simulink model "Model_2_SpeedClosedLoop"  (R2025a)
settings: Solver=VariableStepAuto  StartTime=0.0  StopTime=3  MaxStep=1e-4  RelTol=1e-3  EnableMultiTasking=on
undefined symbols (not defined in the file): Gain_I, Gain_P, Lambda_m, Ld, Lq, Polepairs, Rs, Speed_Gain_I, Speed_Gain_P
libraries: spsControlledVoltageSourceLib x3, slpidlib x3, spsPermanentMagnetSynchronousMachineLib x1, spsGroundLib x1, SignalEditorBlockLib x1, spspowerguiLib x1
settings Model: Creator=dakaihu  LastModifiedBy=ernes
settings SolverCC: AlgebraicLoopSolver=TrustRegion
settings DataIOCC: LimitDataPoints=on  ReturnWorkspaceOutputsName=SDOSimTest_Log
settings OptimizationCC: LifeSpan=inf
settings DebuggingCC: UnconnectedInputMsg=warning  UnconnectedOutputMsg=warning  UnconnectedLineMsg=warning  AllowSymbolicDim=off  SFUnexpectedBacktrackingDiag=warning  SFNoUnconditionalDefaultTransitionDiag=warning  SFExecutionAtInitializationDiag=none  ArithmeticOperatorsInVariantConditions=warning
settings ModelReferenceCC: EnableRefExpFcnMdlSchedulingChecks=on  PropagateSignalLabelsOutOfModel=off
settings SFSimCC: SimUseLocalCustomCode=off  CustomCodeUndefinedFunction=UseInterfaceOnly
settings RTWCC: RTWUseLocalCustomCode=off  GPUComputeCapability=3.5
settings CodeAppCC: StateflowObjectComments=on
settings GRTTargetCC: TargetLangStandard=C89/C90 (ANSI)
settings ConfigComp: CovMetricSettings=dw  CovSaveCumulativeToWorkspaceVar=on  CovSaveSingleToWorkspaceVar=on  CovExternalEMLEnable=off
settings SimscapeCC: SimscapeNormalizeSystem=off

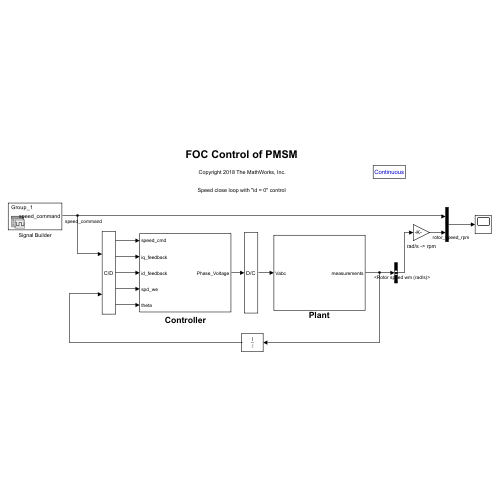
[thumbnail: Simulink's stored preview of the top-level diagram]
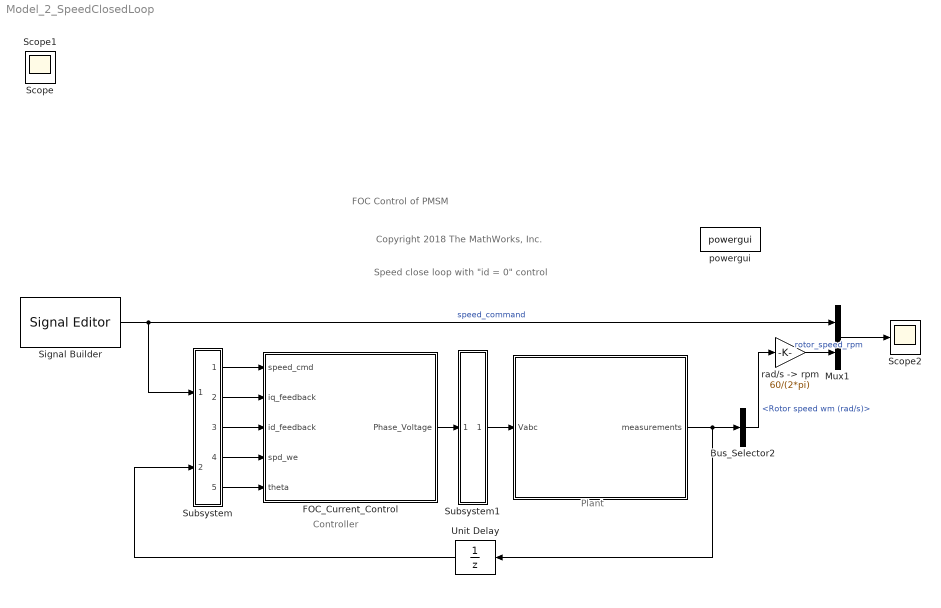
== system Model_2_SpeedClosedLoop ==
  note: Copyright 2018 The MathWorks, Inc.
  note: Speed close loop with "id = 0" control
  note: Controller
  note: Plant
  note: FOC Control of PMSM
  " " : Subsystem
  Bus_Selector2 : BusSelector  OutputSignals=Rotor speed wm (rad/s)
  FOC_Current_Control : Subsystem
  Mux1 : Mux  Inputs=2
  Scope2 : Scope
      settings: ActiveDisplayYMinimum=-125.56583  ActiveDisplayYMaximum=1130.09248
  Signal Builder : SignalEditorBlockLib/Signal Editor  FileName=SignalBuilder.mat  ActiveScenario=Group_1  ActiveSignal=speed_command  IsBus=off  OutputBusObjectStr=Bus: BusObject  SampleTime=0  OutputAfterFinalValue=Extrapolation  Unit=inherit  PreserveSignalName=on  ApplySigPropsToAllScenarios=on  ApplySigPropsToAllSignals=off  SignalPropertySource=Dialog parameters
  Subsystem : Subsystem
      mask Display: fprintf('C/D')
  Subsystem1 : Subsystem
      mask Display: fprintf('D/C')
  Unit Delay : UnitDelay  SampleTime=-1  HasFrameUpgradeWarning=on
  powergui : spspowerguiLib/powergui  SimulationMode=Continuous  SampleTime=1e-5  frequency=60  Iterations=50  frequencyindice=0  Pbase=100e6  ErrMax=1e-4  UnitsV=kV  UnitsW=MW  buscounter=0  FunctionMessages=off  echomessages=off  EnableUseOfTLC=off  CurrentSourceSwitches=off  DisableSnubberDevices=off  DisableRonSwitches=off  DisableVfSwitches=off  DisplayEquations=off  AutomaticDiscreteSolvers=off  SolverType=Tustin/Backward Euler (TBE)  Interpol=off  ExternalGateDelay=off  methode=off  Ts=100  x0status=blocks  SPID=on  SwTol=0  HookPort=off  NonlinearTolerance=1e-4  nMaxIteration=100  ContinueOnMaxIteration=off  RestoreLinks=warning  ResistiveCurrentMeasurement=off  Frange=[0:2:500]  Ylog=off  Xlog=on  ShowGrid=off  save=off  variable=ZData  structure=0  ZoomFFT=on  StartTime=0.0  cycles=1  DisplayStyle=1  fundamental=60  FreqAxis=off  MaxFrequency=1000  frequencyindicesteady=1  RmsSteady=1  display=off
  "rad/s -> rpm" : Gain  Gain=60/(2*pi)
  Scope : Scope
      settings: ActiveDisplayYMinimum=0.10553  ActiveDisplayYMaximum=0.2838
  Scope1 : Scope
      settings: ActiveDisplayYMinimum=-0.03595  ActiveDisplayYMaximum=0.48049  DataLoggingVariableName=ScopeData2
  wires:
  FOC_Current_Control/1(Phase_Voltage) -> Subsystem1/1(In1)
  " "/1(measurements) -> Unit Delay/1, Bus_Selector2/1
  Subsystem1/1(Out1) -> " "/1(Vabc)
  Unit Delay/1 -> Subsystem/2(PMSM_Measurements)
  Signal Builder/1 -> Subsystem/1(speed_cmd), Mux1/1  "speed_command"
  Subsystem/1(Out6) -> FOC_Current_Control/1(speed_cmd)
  Subsystem/2(Out2) -> FOC_Current_Control/2(iq_feedback)
  Subsystem/3(Out3) -> FOC_Current_Control/3(id_feedback)
  Subsystem/4(Out1) -> FOC_Current_Control/4(spd_we)
  Subsystem/5(Out4) -> FOC_Current_Control/5(theta)
  Bus_Selector2/1 -> "rad/s -> rpm"/1  "<Rotor speed wm (rad/s)>"
  "rad/s -> rpm"/1 -> Mux1/2  "rotor_speed_rpm"
  Mux1/1 -> Scope2/1

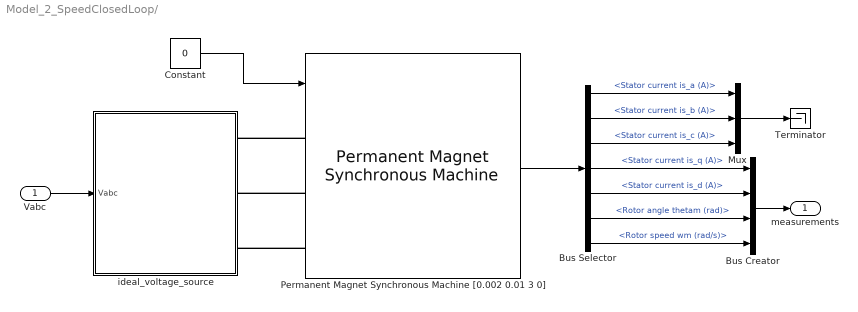
== system Model_2_SpeedClosedLoop/  ==
  Vabc : Inport
  Bus Creator : BusCreator  Inputs=4
  Bus Selector : BusSelector  OutputSignals=Stator current is_a (A),Stator current is_b (A),Stator current is_c (A),Stator current is_q (A),Stator current is_d (A),Rotor angle thetam (rad),Rotor speed wm (rad/s)
  Constant : Constant  Value=0
  Mux : Mux  Inputs=3
  Permanent Magnet Synchronous Machine [0.002 0.01 3 0] : spsPermanentMagnetSynchronousMachineLib/Permanent Magnet Synchronous Machine  NbPhases=3  FluxDistribution=Sinusoidal  RotorType=Salient-pole  MechanicalLoad=Torque Tm  PresetModel=No  ShowDetailedParameters=on  MeasurementBus=off  Resistance=Rs  Inductance=8.5e-3  dqInductances=[Ld,Lq]  La=0.000395  MachineConstant=Flux linkage established by magnets (V.s)  Flux=Lambda_m  VoltageCst=159.9771  TorqueCst=1.323  Flat=120  Mechanical=[0.0027 0.001 4 0]  PolePairs=Polepairs  InitialConditions=[0,0, 0,0]  InitialConditions5ph=[0 0 0 0 0 0]  RefAngle=Aligned with phase A axis (original Park)  IterativeDiscreteModel=Trapezoidal non iterative  TsBlock=-1  TsPowergui=0
  Terminator : Terminator
  ideal_voltage_source : Subsystem  VariantControl=variantPwm == enumPwm.behavior
  measurements : Outport  VectorParamsAs1DForOutWhenUnconnected=off
  wires:
  Vabc/1 -> ideal_voltage_source/1(Vabc)
  Bus Selector/4 -> Bus Creator/1  "<Stator current is_q (A)>"
  Bus Selector/5 -> Bus Creator/2  "<Stator current is_d (A)>"
  Bus Selector/6 -> Bus Creator/3  "<Rotor angle thetam (rad)>"
  Bus Creator/1 -> measurements/1
  Bus Selector/1 -> Mux/1  "<Stator current is_a (A)>"
  Bus Selector/2 -> Mux/2  "<Stator current is_b (A)>"
  Bus Selector/3 -> Mux/3  "<Stator current is_c (A)>"
  Mux/1 -> Terminator/1
  Permanent Magnet Synchronous Machine [0.002 0.01 3 0]/1 -> Bus Selector/1
  Bus Selector/7 -> Bus Creator/4  "<Rotor speed wm (rad/s)>"
  Constant/1 -> Permanent Magnet Synchronous Machine [0.002 0.01 3 0]/1
  connections:
  Permanent Magnet Synchronous Machine [0.002 0.01 3 0]/LConn1 -- ideal_voltage_source/RConn1
  Permanent Magnet Synchronous Machine [0.002 0.01 3 0]/LConn2 -- ideal_voltage_source/RConn2
  Permanent Magnet Synchronous Machine [0.002 0.01 3 0]/LConn3 -- ideal_voltage_source/RConn3

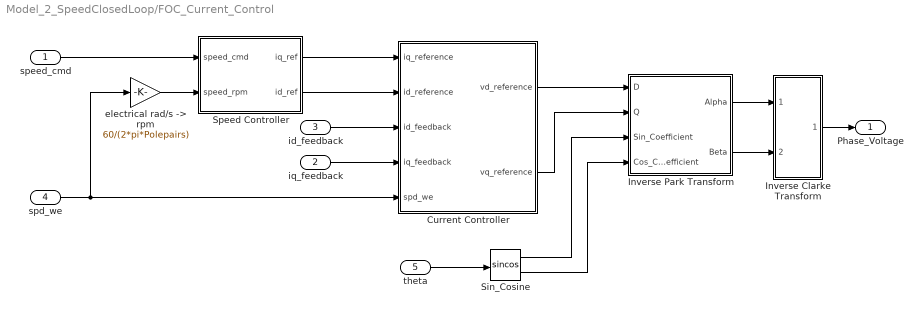
== system Model_2_SpeedClosedLoop/FOC_Current_Control ==
  speed_cmd : Inport
  iq_feedback : Inport  Port=2  SampleTime=1e-4
  id_feedback : Inport  Port=3  SampleTime=1e-4
  spd_we : Inport  Port=4
  theta : Inport  Port=5  SampleTime=1e-4
  Current Controller : Subsystem
  Inverse Clarke Transform : Subsystem
  Inverse Park Transform : Subsystem
  Sin_Cosine : Trigonometry  Operator=sincos
  Speed Controller : Subsystem
  "electrical rad/s -> rpm" : Gain  Gain=60/(2*pi*Polepairs)
  Phase_Voltage : Outport  SampleTime=1e-4  VectorParamsAs1DForOutWhenUnconnected=off
  wires:
  Inverse Clarke Transform/1(ABC) -> Phase_Voltage/1
  Sin_Cosine/2 -> Inverse Park Transform/4(Cos_Coefficient)
  Sin_Cosine/1 -> Inverse Park Transform/3(Sin_Coefficient)
  theta/1 -> Sin_Cosine/1
  Current Controller/2(vq_reference) -> Inverse Park Transform/2(Q)
  Current Controller/1(vd_reference) -> Inverse Park Transform/1(D)
  Inverse Park Transform/1(Alpha) -> Inverse Clarke Transform/1(Alpha)
  Inverse Park Transform/2(Beta) -> Inverse Clarke Transform/2(Beta)
  Speed Controller/1(iq_ref) -> Current Controller/1(iq_reference)
  Speed Controller/2(id_ref) -> Current Controller/2(id_reference)
  id_feedback/1 -> Current Controller/3(id_feedback)
  iq_feedback/1 -> Current Controller/4(iq_feedback)
  spd_we/1 -> "electrical rad/s -> rpm"/1, Current Controller/5(spd_we)
  "electrical rad/s -> rpm"/1 -> Speed Controller/2(speed_rpm)
  speed_cmd/1 -> Speed Controller/1(speed_cmd)

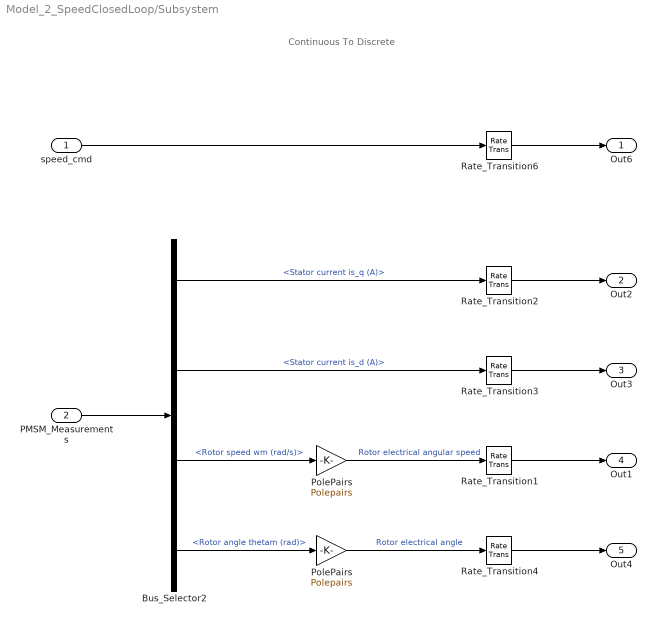
== system Model_2_SpeedClosedLoop/Subsystem ==
  note: Continuous To Discrete
  speed_cmd : Inport
  PMSM_Measurements : Inport  Port=2
  Bus_Selector2 : BusSelector  OutputSignals=Stator current is_q (A),Stator current is_d (A),Rotor speed wm (rad/s),Rotor angle thetam (rad)
  PolePairs : Gain  Gain=Polepairs
  "PolePairs " : Gain  Gain=Polepairs
  Rate_Transition{1..4,6} (5 alike) : RateTransition  Integrity=off  Deterministic=off
  Out6 : Outport  VectorParamsAs1DForOutWhenUnconnected=off
  Out2 : Outport  Port=2  VectorParamsAs1DForOutWhenUnconnected=off
  Out3 : Outport  Port=3  VectorParamsAs1DForOutWhenUnconnected=off
  Out1 : Outport  Port=4  VectorParamsAs1DForOutWhenUnconnected=off
  Out4 : Outport  Port=5  VectorParamsAs1DForOutWhenUnconnected=off
  wires:
  Rate_Transition4/1 -> Out4/1
  Bus_Selector2/2 -> Rate_Transition3/1  "<Stator current is_d (A)>"
  speed_cmd/1 -> Rate_Transition6/1
  Bus_Selector2/1 -> Rate_Transition2/1  "<Stator current is_q (A)>"
  Bus_Selector2/4 -> PolePairs/1  "<Rotor angle thetam (rad)>"
  PMSM_Measurements/1 -> Bus_Selector2/1
  PolePairs/1 -> Rate_Transition4/1  "Rotor electrical angle"
  Rate_Transition6/1 -> Out6/1
  Rate_Transition2/1 -> Out2/1
  Rate_Transition3/1 -> Out3/1
  Rate_Transition1/1 -> Out1/1
  Bus_Selector2/3 -> "PolePairs "/1  "<Rotor speed wm (rad/s)>"
  "PolePairs "/1 -> Rate_Transition1/1  "Rotor electrical angular speed"

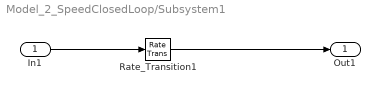
== system Model_2_SpeedClosedLoop/Subsystem1 ==
  In1 : Inport
  Rate_Transition1 : RateTransition  Integrity=off
  Out1 : Outport  VectorParamsAs1DForOutWhenUnconnected=off
  wires:
  In1/1 -> Rate_Transition1/1
  Rate_Transition1/1 -> Out1/1

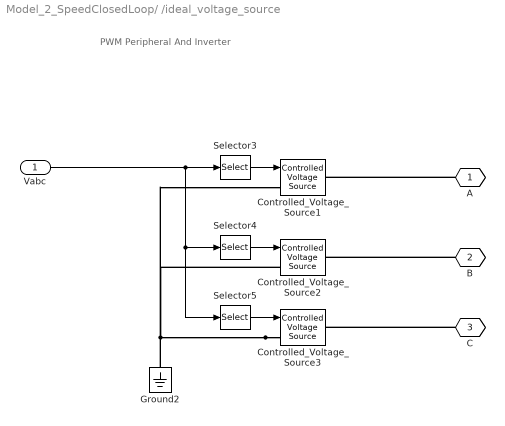
== system Model_2_SpeedClosedLoop/ /ideal_voltage_source ==
  note: PWM Peripheral And Inverter
  Vabc : Inport
  Controlled_Voltage_Source1 : spsControlledVoltageSourceLib/Controlled Voltage Source  Initialize=off  Source_Type=DC  Amplitude=12  Phase=0  Frequency=0  Measurements=None
  Controlled_Voltage_Source2 : spsControlledVoltageSourceLib/Controlled Voltage Source  Initialize=off  Source_Type=DC  Amplitude=12  Phase=0  Frequency=0  Measurements=None
  Controlled_Voltage_Source3 : spsControlledVoltageSourceLib/Controlled Voltage Source  Initialize=off  Source_Type=DC  Amplitude=12  Phase=0  Frequency=0  Measurements=None
  Ground2 : spsGroundLib/Ground  LConnTagsString=a
  Selector3 : Selector  InputPortWidth=3  IndexOptions=Index vector (dialog)  Indices=[1]  OutputSizes=1
  Selector4 : Selector  InputPortWidth=3  IndexOptions=Index vector (dialog)  Indices=2  OutputSizes=1
  Selector5 : Selector  InputPortWidth=3  IndexOptions=Index vector (dialog)  Indices=3  OutputSizes=1
  A : PMIOPort  Tag=PMCPort  Side=Right
  B : PMIOPort  Tag=PMCPort  Port=2  Side=Right
  C : PMIOPort  Tag=PMCPort  Port=3  Side=Right
  wires:
  Vabc/1 -> Selector4/1, Selector5/1, Selector3/1
  Selector5/1 -> Controlled_Voltage_Source3/1
  Selector4/1 -> Controlled_Voltage_Source2/1
  Selector3/1 -> Controlled_Voltage_Source1/1
  connections:
  C/RConn1 -- Controlled_Voltage_Source3/RConn1
  B/RConn1 -- Controlled_Voltage_Source2/RConn1
  A/RConn1 -- Controlled_Voltage_Source1/RConn1
  Controlled_Voltage_Source3/LConn1 -- Controlled_Voltage_Source1/LConn1 -- Controlled_Voltage_Source2/LConn1 -- Ground2/LConn1

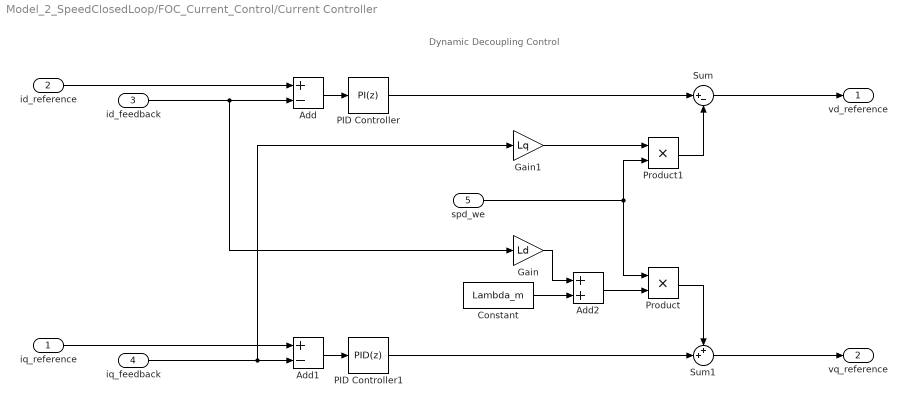
== system Model_2_SpeedClosedLoop/FOC_Current_Control/Current Controller ==
  note: Dynamic Decoupling Control
  iq_reference : Inport  SampleTime=1e-4
  id_reference : Inport  Port=2  SampleTime=1e-4
  id_feedback : Inport  Port=3  SampleTime=1e-4
  iq_feedback : Inport  Port=4  SampleTime=1e-4
  spd_we : Inport  Port=5  SampleTime=1e-4
  Add : Sum  Inputs=+-
  Add1 : Sum  Inputs=+-
  Add2 : Sum
  Constant : Constant  Value=Lambda_m  SampleTime=1e-4
  Gain : Gain  Gain=Ld
  Gain1 : Gain  Gain=Lq
  PID Controller : slpidlib/PID Controller  Controller=PI  Form=Parallel  TimeDomain=Discrete-time  UseExternalTs=off  SampleTime=-1  IntegratorMethod=Forward Euler  FilterMethod=Forward Euler  ControllerParametersSource=internal  P=Gain_P  I=Gain_I  UseKiTs=off  D=0  UseExternalDerivativeSource=off  N=100  UseFilter=on  TunerSelectOption=Transfer Function Based (PID Tuner App)  InitialConditionSource=internal  InitialConditionForIntegrator=0  InitialConditionForFilter=0  DifferentiatorICPrevScaledInput=0  ExternalReset=none  TrackingMode=off  Kt=1  LimitOutput=off  SatLimitsSource=internal  UpperSaturationLimit=inf  LowerSaturationLimit=-inf  LinearizeAsGain=on  AntiWindupMode=none  Kb=1  LimitIntegrator=off  UpperIntegratorSaturationLimit=inf  LowerIntegratorSaturationLimit=-inf  POutMin=[]  POutMax=[]  IOutMin=[]  IOutMax=[]  DOutMin=[]  DOutMax=[]  NOutMin=[]  NOutMax=[]  SumOutMin=[]  SumOutMax=[]  SaturationOutMin=[]  SaturationOutMax=[]  PParamMin=[]  PParamMax=[]  IParamMin=[]  IParamMax=[]  DParamMin=[]  DParamMax=[]  NParamMin=[]  NParamMax=[]  KbParamMin=[]  KbParamMax=[]  KtParamMin=[]  KtParamMax=[]  KbOutMin=[]  KbOutMax=[]  KtOutMin=[]  KtOutMax=[]  IntegratorOutMin=[]  IntegratorOutMax=[]  FilterOutMin=[]  FilterOutMax=[]  SumI1OutMin=[]  SumI1OutMax=[]  SumI2OutMin=[]  SumI2OutMax=[]  SumI3OutMin=[]  SumI3OutMax=[]  SumI4OutMin=[]  SumI4OutMax=[]  SumDOutMin=[]  SumDOutMax=[]  DifferentiatorOutMin=[]  DifferentiatorOutMax=[]  FilterDiffOutCoefMin=[]  FilterDiffOutCoefMax=[]  ReciprocalOutMin=[]  ReciprocalOutMax=[]  SumDenOutMin=[]  SumDenOutMax=[]  SumNumOutMin=[]  SumNumOutMax=[]  DivideOutMin=[]  DivideOutMax=[]  UdiffTsProdOutMin=[]  UdiffTsProdOutMax=[]  NTsProdOutMin=[]  NTsProdOutMax=[]  UintegralTsProdOutMin=[]  UintegralTsProdOutMax=[]  UngainTsProdOutMin=[]  UngainTsProdOutMax=[]  ClampingZeroOutDataTypeStr=Inherit: Inherit via back propagation  ClampingZeroOutMin=[]  ClampingZeroOutMax=[]  FilterDenConstantOutDataTypeStr=Inherit: Inherit via back propagation  FilterDenConstantOutMin=[]  FilterDenConstantOutMax=[]  PCopyOutDataTypeStr=Inherit: Inherit via back propagation  PCopyOutMin=[]  PCopyOutMax=[]  NCopyOutDataTypeStr=Inherit: Inherit via back propagation  NCopyOutMin=[]  NCopyOutMax=[]  IntegratorContinuousStateAttributes=''  IntegratorStateMustResolveToSignalObject=off  IntegratorRTWStateStorageClass=Auto  FilterContinuousStateAttributes=''  FilterStateMustResolveToSignalObject=off  FilterRTWStateStorageClass=Auto  ParallelPVariant=InternalParameters  IdealPVariant=Disabled  IVariant=InternalParameters  DVariant=Disabled  IntegratorVariant=Discrete  SatVariant=Disabled  AWVariant=Passthrough  PCopyVariant=Disabled  TRVariant=Disabled  FdbkBlocksVariant=Forward  IdealPFdbkVariant=Disabled  SatFdbkVariant=Disabled  DerivativeFilterVariant=Disabled  NVariant=Disabled  NCopyVariant=Disabled_SignalSpec  FilterICVariant=Disabled  IntegratorICVariant=InternalICs  ExternalResetVariant=Disabled  TRSumVariant=Passthrough  SumFdbkVariant=Disabled  SumVariant=Sum_PI  TsampFilterVariant=InternalTs  TsampNgainVariant=Passthrough  TsampIntegralVariant=Disabled_SignalSpec  ExternalSaturationOutDataTypeStr=Inherit: Same as second input  DerivativeSourceVariant=Disabled  PreIntVariant=InternalPreInt
  PID Controller1 : slpidlib/PID Controller  Controller=PID  Form=Parallel  TimeDomain=Discrete-time  UseExternalTs=off  SampleTime=-1  IntegratorMethod=Forward Euler  FilterMethod=Forward Euler  ControllerParametersSource=internal  P=Gain_P  I=Gain_I  UseKiTs=off  D=0  UseExternalDerivativeSource=off  N=100  UseFilter=on  TunerSelectOption=Transfer Function Based (PID Tuner App)  InitialConditionSource=internal  InitialConditionForIntegrator=0  InitialConditionForFilter=0  DifferentiatorICPrevScaledInput=0  ExternalReset=none  TrackingMode=off  Kt=1  LimitOutput=off  SatLimitsSource=internal  UpperSaturationLimit=inf  LowerSaturationLimit=-inf  LinearizeAsGain=on  AntiWindupMode=none  Kb=1  LimitIntegrator=off  UpperIntegratorSaturationLimit=inf  LowerIntegratorSaturationLimit=-inf  POutMin=[]  POutMax=[]  IOutMin=[]  IOutMax=[]  DOutMin=[]  DOutMax=[]  NOutMin=[]  NOutMax=[]  SumOutMin=[]  SumOutMax=[]  SaturationOutMin=[]  SaturationOutMax=[]  PParamMin=[]  PParamMax=[]  IParamMin=[]  IParamMax=[]  DParamMin=[]  DParamMax=[]  NParamMin=[]  NParamMax=[]  KbParamMin=[]  KbParamMax=[]  KtParamMin=[]  KtParamMax=[]  KbOutMin=[]  KbOutMax=[]  KtOutMin=[]  KtOutMax=[]  IntegratorOutMin=[]  IntegratorOutMax=[]  FilterOutMin=[]  FilterOutMax=[]  SumI1OutMin=[]  SumI1OutMax=[]  SumI2OutMin=[]  SumI2OutMax=[]  SumI3OutMin=[]  SumI3OutMax=[]  SumI4OutMin=[]  SumI4OutMax=[]  SumDOutMin=[]  SumDOutMax=[]  DifferentiatorOutMin=[]  DifferentiatorOutMax=[]  FilterDiffOutCoefMin=[]  FilterDiffOutCoefMax=[]  ReciprocalOutMin=[]  ReciprocalOutMax=[]  SumDenOutMin=[]  SumDenOutMax=[]  SumNumOutMin=[]  SumNumOutMax=[]  DivideOutMin=[]  DivideOutMax=[]  UdiffTsProdOutMin=[]  UdiffTsProdOutMax=[]  NTsProdOutMin=[]  NTsProdOutMax=[]  UintegralTsProdOutMin=[]  UintegralTsProdOutMax=[]  UngainTsProdOutMin=[]  UngainTsProdOutMax=[]  ClampingZeroOutDataTypeStr=Inherit: Inherit via back propagation  ClampingZeroOutMin=[]  ClampingZeroOutMax=[]  FilterDenConstantOutDataTypeStr=Inherit: Inherit via back propagation  FilterDenConstantOutMin=[]  FilterDenConstantOutMax=[]  PCopyOutDataTypeStr=Inherit: Inherit via back propagation  PCopyOutMin=[]  PCopyOutMax=[]  NCopyOutDataTypeStr=Inherit: Inherit via back propagation  NCopyOutMin=[]  NCopyOutMax=[]  IntegratorContinuousStateAttributes=''  IntegratorStateMustResolveToSignalObject=off  IntegratorRTWStateStorageClass=Auto  FilterContinuousStateAttributes=''  FilterStateMustResolveToSignalObject=off  FilterRTWStateStorageClass=Auto  ParallelPVariant=InternalParameters  IdealPVariant=Disabled  IVariant=InternalParameters  DVariant=InternalParameters  IntegratorVariant=Discrete  SatVariant=Disabled  AWVariant=Passthrough  PCopyVariant=Disabled  TRVariant=Disabled  FdbkBlocksVariant=Forward  IdealPFdbkVariant=Disabled  SatFdbkVariant=Disabled  DerivativeFilterVariant=ForwardEulerFilter  NVariant=InternalParameters  NCopyVariant=Disabled  FilterICVariant=InternalICsFilter  IntegratorICVariant=InternalICs  ExternalResetVariant=Disabled  TRSumVariant=Passthrough  SumFdbkVariant=Disabled  SumVariant=Sum_PID  TsampFilterVariant=InternalTs  TsampNgainVariant=Passthrough  TsampIntegralVariant=Disabled_SignalSpec  ExternalSaturationOutDataTypeStr=Inherit: Same as second input  DerivativeSourceVariant=ErrorSignal  PreIntVariant=InternalPreInt
  Product : Product
  Product1 : Product
  Sum : Sum  Inputs=|+-
  Sum1 : Sum  Inputs=++|
  vd_reference : Outport  SampleTime=1e-4  VectorParamsAs1DForOutWhenUnconnected=off
  vq_reference : Outport  Port=2  SampleTime=1e-4  VectorParamsAs1DForOutWhenUnconnected=off
  wires:
  Sum/1 -> vd_reference/1
  PID Controller/1 -> Sum/1
  id_feedback/1 -> Gain/1, Add/2
  Add/1 -> PID Controller/1
  iq_feedback/1 -> Gain1/1, Add1/2
  id_reference/1 -> Add/1
  Add1/1 -> PID Controller1/1
  iq_reference/1 -> Add1/1
  Sum1/1 -> vq_reference/1
  PID Controller1/1 -> Sum1/2
  Gain/1 -> Add2/1
  Constant/1 -> Add2/2
  Add2/1 -> Product/2
  spd_we/1 -> Product1/2, Product/1
  Gain1/1 -> Product1/1
  Product1/1 -> Sum/2
  Product/1 -> Sum1/1

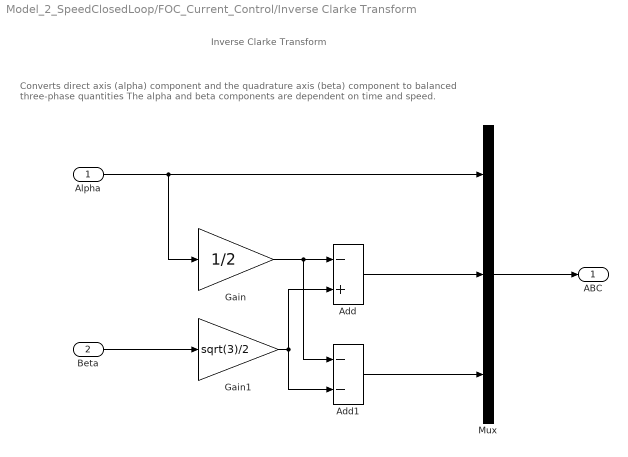
== system Model_2_SpeedClosedLoop/FOC_Current_Control/Inverse Clarke Transform ==
  note: Inverse Clarke Transform
  note: Converts direct axis (alpha) component and the quadrature axis (beta) component to balanced three-phase quantities
      | The alpha and beta components are dependent on time and speed.
  Alpha : Inport
  Beta : Inport  Port=2
  Add : Sum  Inputs=-+  OutDataTypeStr=Inherit: Same as first input
  Add1 : Sum  Inputs=--  OutDataTypeStr=Inherit: Same as first input
  Gain : Gain  Gain=1/2
  Gain1 : Gain  Gain=sqrt(3)/2
  Mux : Mux  Inputs=3
  ABC : Outport  VectorParamsAs1DForOutWhenUnconnected=off
  wires:
  Beta/1 -> Gain1/1
  Mux/1 -> ABC/1
  Alpha/1 -> Mux/1, Gain/1
  Add1/1 -> Mux/3
  Gain1/1 -> Add1/2, Add/2
  Gain/1 -> Add1/1, Add/1
  Add/1 -> Mux/2

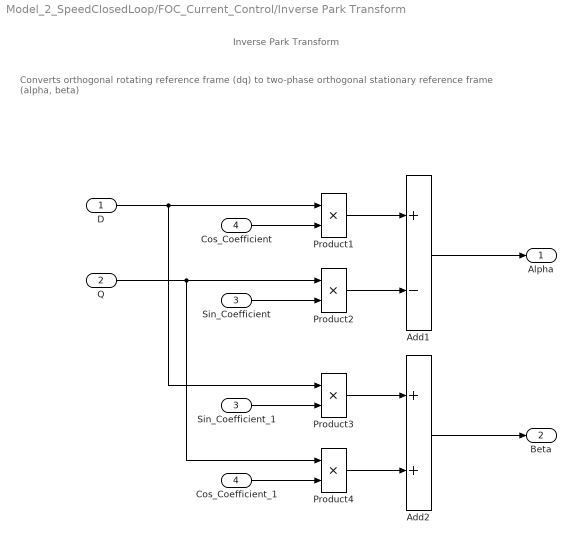
== system Model_2_SpeedClosedLoop/FOC_Current_Control/Inverse Park Transform ==
  note: Converts orthogonal rotating reference frame (dq) to two-phase orthogonal stationary reference frame (alpha, beta)
  note: Inverse Park Transform
  D : Inport
  Q : Inport  Port=2
  Sin_Coefficient : Inport  Port=3
  Cos_Coefficient : Inport  Port=4
  Add1 : Sum  Inputs=+-  OutDataTypeStr=Inherit: Same as first input
  Add2 : Sum  OutDataTypeStr=Inherit: Same as first input
  Cos_Coefficient_1 : InportShadow  Port=4
  Product{1..4} (4 alike) : Product  RndMeth=Simplest
  Sin_Coefficient_1 : InportShadow  Port=3
  Alpha : Outport  VectorParamsAs1DForOutWhenUnconnected=off
  Beta : Outport  Port=2  VectorParamsAs1DForOutWhenUnconnected=off
  wires:
  Sin_Coefficient_1/1 -> Product3/2
  Product2/1 -> Add1/2
  Cos_Coefficient_1/1 -> Product4/2
  Add2/1 -> Beta/1
  Product3/1 -> Add2/1
  Add1/1 -> Alpha/1
  Product1/1 -> Add1/1
  Product4/1 -> Add2/2
  Sin_Coefficient/1 -> Product2/2
  D/1 -> Product3/1, Product1/1
  Q/1 -> Product2/1, Product4/1
  Cos_Coefficient/1 -> Product1/2

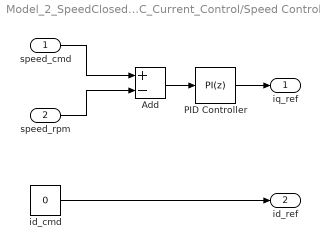
== system Model_2_SpeedClosedLoop/FOC_Current_Control/Speed Controller ==
  speed_cmd : Inport  SampleTime=1e-3
  speed_rpm : Inport  Port=2  SampleTime=1e-3
  Add : Sum  Inputs=+-
  PID Controller : slpidlib/PID Controller  Controller=PI  Form=Parallel  TimeDomain=Discrete-time  UseExternalTs=off  SampleTime=-1  IntegratorMethod=Forward Euler  FilterMethod=Forward Euler  ControllerParametersSource=internal  P=Speed_Gain_P  I=Speed_Gain_I  UseKiTs=off  D=0  UseExternalDerivativeSource=off  N=100  UseFilter=on  TunerSelectOption=Transfer Function Based (PID Tuner App)  InitialConditionSource=internal  InitialConditionForIntegrator=0  InitialConditionForFilter=0  DifferentiatorICPrevScaledInput=0  ExternalReset=none  TrackingMode=off  Kt=1  LimitOutput=off  SatLimitsSource=internal  UpperSaturationLimit=inf  LowerSaturationLimit=-inf  LinearizeAsGain=on  AntiWindupMode=none  Kb=1  LimitIntegrator=off  UpperIntegratorSaturationLimit=inf  LowerIntegratorSaturationLimit=-inf  POutMin=[]  POutMax=[]  IOutMin=[]  IOutMax=[]  DOutMin=[]  DOutMax=[]  NOutMin=[]  NOutMax=[]  SumOutMin=[]  SumOutMax=[]  SaturationOutMin=[]  SaturationOutMax=[]  PParamMin=[]  PParamMax=[]  IParamMin=[]  IParamMax=[]  DParamMin=[]  DParamMax=[]  NParamMin=[]  NParamMax=[]  KbParamMin=[]  KbParamMax=[]  KtParamMin=[]  KtParamMax=[]  KbOutMin=[]  KbOutMax=[]  KtOutMin=[]  KtOutMax=[]  IntegratorOutMin=[]  IntegratorOutMax=[]  FilterOutMin=[]  FilterOutMax=[]  SumI1OutMin=[]  SumI1OutMax=[]  SumI2OutMin=[]  SumI2OutMax=[]  SumI3OutMin=[]  SumI3OutMax=[]  SumI4OutMin=[]  SumI4OutMax=[]  SumDOutMin=[]  SumDOutMax=[]  DifferentiatorOutMin=[]  DifferentiatorOutMax=[]  FilterDiffOutCoefMin=[]  FilterDiffOutCoefMax=[]  ReciprocalOutMin=[]  ReciprocalOutMax=[]  SumDenOutMin=[]  SumDenOutMax=[]  SumNumOutMin=[]  SumNumOutMax=[]  DivideOutMin=[]  DivideOutMax=[]  UdiffTsProdOutMin=[]  UdiffTsProdOutMax=[]  NTsProdOutMin=[]  NTsProdOutMax=[]  UintegralTsProdOutMin=[]  UintegralTsProdOutMax=[]  UngainTsProdOutMin=[]  UngainTsProdOutMax=[]  ClampingZeroOutDataTypeStr=Inherit: Inherit via back propagation  ClampingZeroOutMin=[]  ClampingZeroOutMax=[]  FilterDenConstantOutDataTypeStr=Inherit: Inherit via back propagation  FilterDenConstantOutMin=[]  FilterDenConstantOutMax=[]  PCopyOutDataTypeStr=Inherit: Inherit via back propagation  PCopyOutMin=[]  PCopyOutMax=[]  NCopyOutDataTypeStr=Inherit: Inherit via back propagation  NCopyOutMin=[]  NCopyOutMax=[]  IntegratorContinuousStateAttributes=''  IntegratorStateMustResolveToSignalObject=off  IntegratorRTWStateStorageClass=Auto  FilterContinuousStateAttributes=''  FilterStateMustResolveToSignalObject=off  FilterRTWStateStorageClass=Auto  ParallelPVariant=InternalParameters  IdealPVariant=Disabled  IVariant=InternalParameters  DVariant=Disabled  IntegratorVariant=Discrete  SatVariant=Disabled  AWVariant=Passthrough  PCopyVariant=Disabled  TRVariant=Disabled  FdbkBlocksVariant=Forward  IdealPFdbkVariant=Disabled  SatFdbkVariant=Disabled  DerivativeFilterVariant=Disabled  NVariant=Disabled  NCopyVariant=Disabled_SignalSpec  FilterICVariant=Disabled  IntegratorICVariant=InternalICs  ExternalResetVariant=Disabled  TRSumVariant=Passthrough  SumFdbkVariant=Disabled  SumVariant=Sum_PI  TsampFilterVariant=InternalTs  TsampNgainVariant=Passthrough  TsampIntegralVariant=Disabled_SignalSpec  ExternalSaturationOutDataTypeStr=Inherit: Same as second input  DerivativeSourceVariant=Disabled  PreIntVariant=InternalPreInt
  id_cmd : Constant  Value=0  SampleTime=1e-3
  iq_ref : Outport  VectorParamsAs1DForOutWhenUnconnected=off
  id_ref : Outport  Port=2  VectorParamsAs1DForOutWhenUnconnected=off
  wires:
  id_cmd/1 -> id_ref/1
  PID Controller/1 -> iq_ref/1
  Add/1 -> PID Controller/1
  speed_cmd/1 -> Add/1
  speed_rpm/1 -> Add/2
